simulink library "full_bridge_zvs_pwm_modulator"  (R2026a)
settings: Solver=VariableStepAuto
undefined symbols (not defined in the file): dead_time_DAB, fPWM_DAB, tc, TRGO_double_update
settings Model: Creator=dbagn  LastModifiedBy=dbagn

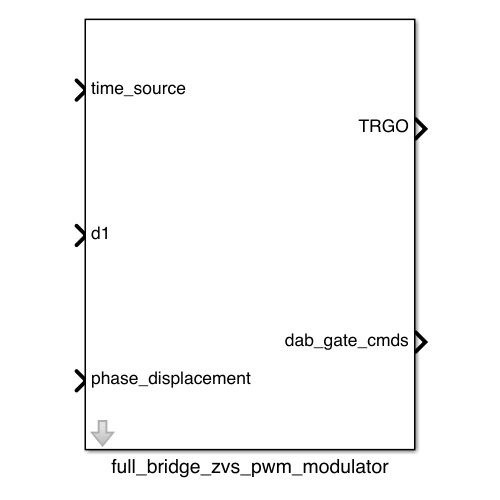
[thumbnail: Simulink's stored preview of the top-level diagram]
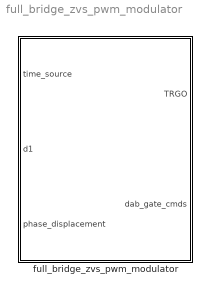
== system full_bridge_zvs_pwm_modulator ==
  full_bridge_zvs_pwm_modulator : Subsystem  mask{fPWM_m=fPWM_DAB, m_up_m=1, m_low_m=0, dead_time_DAB_m=dead_time_DAB, pos_cmd_gate_m=18, neg_cmd_gate_m=-3, polarity_m=1, tc_m=tc, max_phase_displacement_m=pi, trgo_double_update_m=TRGO_double_update}
      mask prompts: fPWM_m "PWM Frequency (Hz)"; m_up_m "Max Input Modulation Value"; m_low_m "Min Input Modulation Value"; dead_time_DAB_m "Dead Time (s)"; pos_cmd_gate_m "Positive Gate Voltage cmd (V)"; neg_cmd_gate_m "Negative Gate Voltage cmd (V)"; polarity_m "Polarity (pu)"; tc_m "Sampling time"; max_phase_displacement_m "Max Phase Displacement"; trgo_double_update_m "TRGO double update"

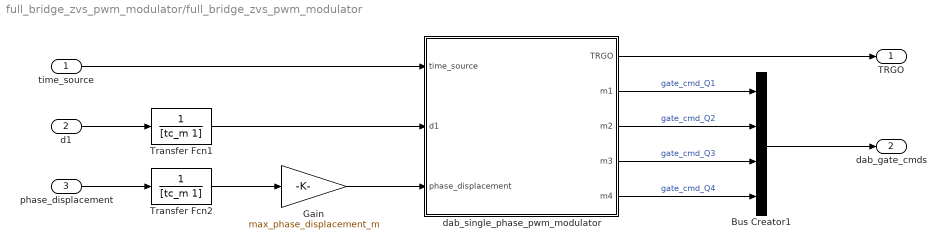
== system full_bridge_zvs_pwm_modulator/full_bridge_zvs_pwm_modulator ==
  time_source : Inport
  d1 : Inport  Port=2
  phase_displacement : Inport  Port=3
  Bus Creator1 : BusCreator  Inputs=4
  Gain : Gain  Gain=max_phase_displacement_m  OutDataTypeStr=double
  Transfer Fcn1 : TransferFcn  Denominator=[tc_m 1]
  Transfer Fcn2 : TransferFcn  Denominator=[tc_m 1]
  dab_single_phase_pwm_modulator : Subsystem  mask{f=fPWM_m, m_up=m_up_m, m_low=m_low_m, dead_time=dead_time_DAB_m, pos_cmd_gate=pos_cmd_gate_m, neg_cmd_gate=neg_cmd_gate_m, polarity=polarity_m, trgo_double_update=trgo_double_update_m}
      mask prompts: f "Frequency (Hz)"; m_up "Max Input Modulation Value"; m_low "Min Input Modulation Value"; dead_time "Dead Time (s)"; pos_cmd_gate "Positive Gate Voltage (V)"; neg_cmd_gate "Negative Gate Voltage (V)"; polarity "Polarity (pu)"; trgo_double_update "TRGO double update"
  TRGO : Outport
  dab_gate_cmds : Outport  Port=2
  wires:
  Bus Creator1/1 -> dab_gate_cmds/1
  dab_single_phase_pwm_modulator/5(m4) -> Bus Creator1/4  "gate_cmd_Q4"
  dab_single_phase_pwm_modulator/4(m3) -> Bus Creator1/3  "gate_cmd_Q3"
  dab_single_phase_pwm_modulator/3(m2) -> Bus Creator1/2  "gate_cmd_Q2"
  dab_single_phase_pwm_modulator/2(m1) -> Bus Creator1/1  "gate_cmd_Q1"
  Transfer Fcn2/1 -> Gain/1
  Transfer Fcn1/1 -> dab_single_phase_pwm_modulator/2(d1)
  dab_single_phase_pwm_modulator/1(TRGO) -> TRGO/1
  time_source/1 -> dab_single_phase_pwm_modulator/1(time_source)
  Gain/1 -> dab_single_phase_pwm_modulator/3(phase_displacement)
  phase_displacement/1 -> Transfer Fcn2/1
  d1/1 -> Transfer Fcn1/1

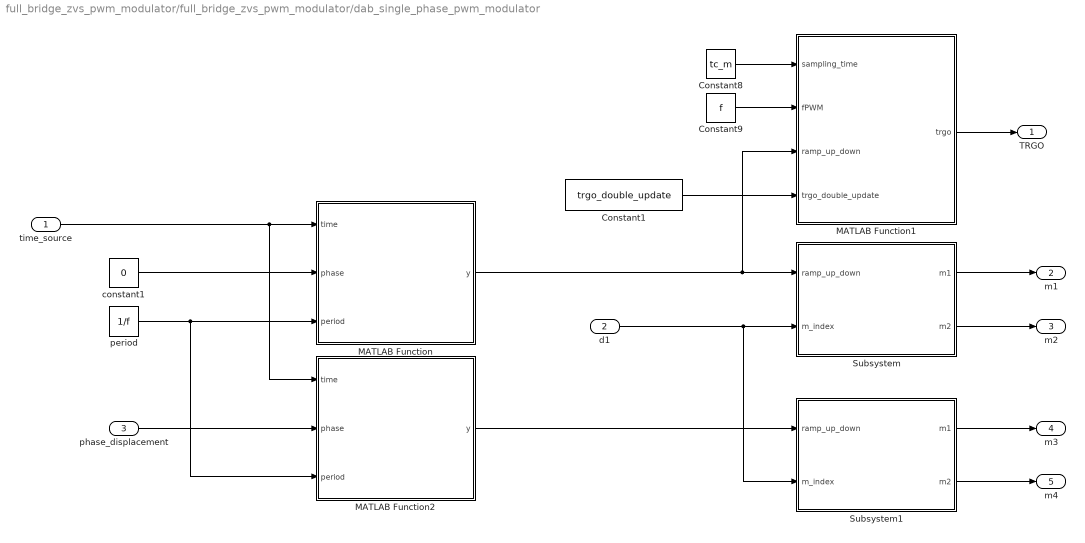
== system full_bridge_zvs_pwm_modulator/full_bridge_zvs_pwm_modulator/dab_single_phase_pwm_modulator ==
  time_source : Inport
  d1 : Inport  Port=2
  phase_displacement : Inport  Port=3
  Constant1 : Constant  Value=trgo_double_update
  Constant8 : Constant  Value=tc_m
  Constant9 : Constant  Value=f
  MATLAB Function : MATLAB Function  TreatAsAtomicUnit=on  SystemSampleTime=tc_m
  MATLAB Function1 : MATLAB Function  TreatAsAtomicUnit=on  SystemSampleTime=tc_m
  MATLAB Function2 : MATLAB Function  TreatAsAtomicUnit=on  SystemSampleTime=tc_m
  Subsystem : Subsystem
  Subsystem1 : Subsystem
  constant1 : Constant  Value=0
  period : Constant  Value=1/f
  TRGO : Outport
  m1 : Outport  Port=2
  m2 : Outport  Port=3
  m3 : Outport  Port=4
  m4 : Outport  Port=5
  wires:
  Constant1/1 -> MATLAB Function1/4(trgo_double_update)
  d1/1 -> Subsystem1/2(m_index), Subsystem/2(m_index)
  time_source/1 -> MATLAB Function2/1(time), MATLAB Function/1(time)
  period/1 -> MATLAB Function2/3(period), MATLAB Function/3(period)
  phase_displacement/1 -> MATLAB Function2/2(phase)
  MATLAB Function2/1(y) -> Subsystem1/1(ramp_up_down)
  Subsystem1/1(m1) -> m3/1
  Subsystem1/2(m2) -> m4/1
  Subsystem/2(m2) -> m2/1
  Subsystem/1(m1) -> m1/1
  constant1/1 -> MATLAB Function/2(phase)
  Constant9/1 -> MATLAB Function1/2(fPWM)
  MATLAB Function1/1(trgo) -> TRGO/1
  Constant8/1 -> MATLAB Function1/1(sampling_time)
  MATLAB Function/1(y) -> MATLAB Function1/3(ramp_up_down), Subsystem/1(ramp_up_down)

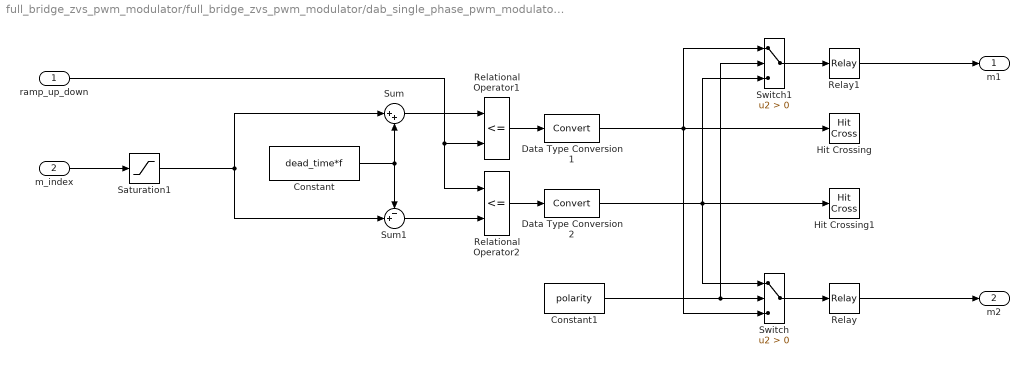
== system full_bridge_zvs_pwm_modulator/full_bridge_zvs_pwm_modulator/dab_single_phase_pwm_modulator/Subsystem ==
  ramp_up_down : Inport
  m_index : Inport  Port=2
  Constant : Constant  Value=dead_time*f
  Constant1 : Constant  Value=polarity
  Data Type Conversion1 : DataTypeConversion
  Data Type Conversion2 : DataTypeConversion
  Hit Crossing : HitCross  ShowOutputPort=off
  Hit Crossing1 : HitCross  ShowOutputPort=off
  Relational Operator1 : RelationalOperator  Operator=<=  InputSameDT=off
  Relational Operator2 : RelationalOperator  Operator=<=  InputSameDT=off
  Relay : Relay  OnOutputValue=pos_cmd_gate  OffOutputValue=neg_cmd_gate
  Relay1 : Relay  OnOutputValue=pos_cmd_gate  OffOutputValue=neg_cmd_gate
  Saturation1 : Saturate  UpperLimit=m_up  LowerLimit=m_low
  Sum : Sum  Inputs=|++  SaturateOnIntegerOverflow=on
  Sum1 : Sum  Inputs=-+|  SaturateOnIntegerOverflow=on
  Switch : Switch  Criteria=u2 > Threshold  SaturateOnIntegerOverflow=off  InputSameDT=off
  Switch1 : Switch  Criteria=u2 > Threshold  SaturateOnIntegerOverflow=off  InputSameDT=off
  m1 : Outport
  m2 : Outport  Port=2
  wires:
  Switch/1 -> Relay/1
  Sum/1 -> Relational Operator1/1
  Sum1/1 -> Relational Operator2/2
  Data Type Conversion1/1 -> Switch1/1, Switch/3, Hit Crossing/1
  Relay1/1 -> m1/1
  Relay/1 -> m2/1
  Relational Operator1/1 -> Data Type Conversion1/1
  m_index/1 -> Saturation1/1
  Constant1/1 -> Switch/2, Switch1/2
  Switch1/1 -> Relay1/1
  ramp_up_down/1 -> Relational Operator1/2, Relational Operator2/1
  Constant/1 -> Sum1/1, Sum/2
  Relational Operator2/1 -> Data Type Conversion2/1
  Saturation1/1 -> Sum1/2, Sum/1
  Data Type Conversion2/1 -> Hit Crossing1/1, Switch1/3, Switch/1

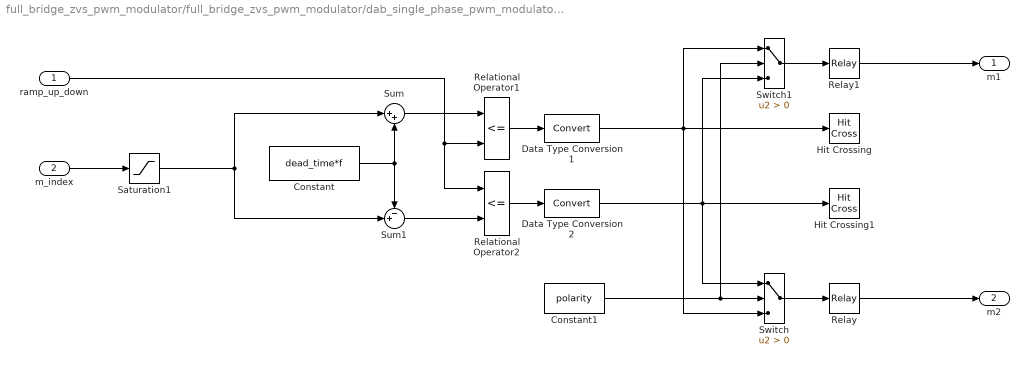
== system full_bridge_zvs_pwm_modulator/full_bridge_zvs_pwm_modulator/dab_single_phase_pwm_modulator/Subsystem1 ==
  ramp_up_down : Inport
  m_index : Inport  Port=2
  Constant : Constant  Value=dead_time*f
  Constant1 : Constant  Value=polarity
  Data Type Conversion1 : DataTypeConversion
  Data Type Conversion2 : DataTypeConversion
  Hit Crossing : HitCross  ShowOutputPort=off
  Hit Crossing1 : HitCross  ShowOutputPort=off
  Relational Operator1 : RelationalOperator  Operator=<=  InputSameDT=off
  Relational Operator2 : RelationalOperator  Operator=<=  InputSameDT=off
  Relay : Relay  OnOutputValue=pos_cmd_gate  OffOutputValue=neg_cmd_gate
  Relay1 : Relay  OnOutputValue=pos_cmd_gate  OffOutputValue=neg_cmd_gate
  Saturation1 : Saturate  UpperLimit=m_up  LowerLimit=m_low
  Sum : Sum  Inputs=|++  SaturateOnIntegerOverflow=on
  Sum1 : Sum  Inputs=-+|  SaturateOnIntegerOverflow=on
  Switch : Switch  Criteria=u2 > Threshold  SaturateOnIntegerOverflow=off  InputSameDT=off
  Switch1 : Switch  Criteria=u2 > Threshold  SaturateOnIntegerOverflow=off  InputSameDT=off
  m1 : Outport
  m2 : Outport  Port=2
  wires:
  Data Type Conversion2/1 -> Switch/1, Switch1/3, Hit Crossing1/1
  Saturation1/1 -> Sum/1, Sum1/2
  Relational Operator2/1 -> Data Type Conversion2/1
  Constant/1 -> Sum/2, Sum1/1
  ramp_up_down/1 -> Relational Operator2/1, Relational Operator1/2
  Switch1/1 -> Relay1/1
  Constant1/1 -> Switch1/2, Switch/2
  m_index/1 -> Saturation1/1
  Relational Operator1/1 -> Data Type Conversion1/1
  Relay/1 -> m2/1
  Relay1/1 -> m1/1
  Data Type Conversion1/1 -> Hit Crossing/1, Switch/3, Switch1/1
  Sum1/1 -> Relational Operator2/2
  Sum/1 -> Relational Operator1/1
  Switch/1 -> Relay/1

== matlab function full_bridge_zvs_pwm_modulator/dab_single_phase_pwm_modulator/MATLAB Function2 ==
  data: time input; y output; phase input; period input
function y = ramp_up_down(time,phase,period)
x = sin(2*pi/period*time - phase -pi/2);
y = asin(x)/pi + 1/2;

== matlab function full_bridge_zvs_pwm_modulator/dab_single_phase_pwm_modulator/MATLAB Function ==
  data: time input; y output; phase input; period input
function y = ramp_up_down(time,phase,period)
x = sin(2*pi/period*time - phase -pi/2);
y = asin(x)/pi + 1/2;

== matlab function full_bridge_zvs_pwm_modulator/dab_single_phase_pwm_modulator/MATLAB Function1 ==
  data: sampling_time input; fPWM input; ramp_up_down input; trgo output; trgo_double_update input
function trgo = trgo_gen(sampling_time,fPWM, ramp_up_down, trgo_double_update)

th = fPWM*sampling_time*2;

if trgo_double_update
    if (((ramp_up_down >= 0) && (ramp_up_down <= th)) || ...
            ((ramp_up_down <= 1) && (ramp_up_down >= 1-th)))
        trgo = 1;
    else
        trgo = 0;
    end
else
    if ((ramp_up_down >= 0) && (ramp_up_down <= th))
        trgo = 1;
    else
        trgo = 0;
    end
end
